simulink model "Gearbox_SLX"  (R2019b)
settings: Solver=VariableStepAuto  StartTime=0.0  StopTime=10.0  RelTol=1e-3
values from neighbouring files (symbols this model uses):
  b_mc = 1*(Nm/rad)    (= 1)    [Gearbox_SLX_m.m]
  J_mc = 1*kg*meters^2    (= 1)    [Gearbox_SLX_m.m]
  K_c = 10^7*(Newton/meters)    (= 10000000)    [Gearbox_SLX_m.m]
  P_2_0 = 0    [Gearbox_SLX_m.m]
  r_1 = 1*cm    (= 0.01)    [Gearbox_SLX_m.m]
  r_2 = 9.7*cm    (= 0.097)    [Gearbox_SLX_m.m]
  T_m_0 = 20*Nm    (= 20)    [Gearbox_SLX_m.m]
  Ts = Tfin/Nr_Ts_Points    (= 0.0025)    [Gearbox_SLX_m.m]
  W_w_0 = 0*Nm    (= 0)    [Gearbox_SLX_m.m]
  x_5_0 = 0    [Gearbox_SLX_m.m]
settings Model: Creator=Luca  LastModifiedBy=giaco
settings DataIOCC: ReturnWorkspaceOutputs=off
settings DebuggingCC: ArithmeticOperatorsInVariantConditions=warning
settings SFSimCC: SimUseLocalCustomCode=off  CustomCodeUndefinedFunction=UseInterfaceOnly
settings RTWCC: RTWUseLocalCustomCode=off

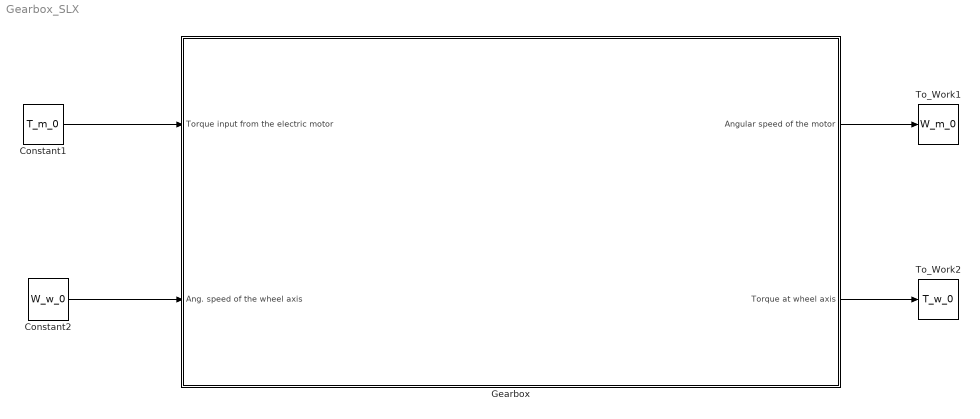
== system Gearbox_SLX ==
  Constant1 : Constant  Value=T_m_0
  Constant2 : Constant  Value=W_w_0
  Gearbox : Subsystem
  To_Work1 : ToWorkspace  VariableName=W_m_0  SampleTime=Ts
      settings: MaxDataPoints=10000
  To_Work2 : ToWorkspace  VariableName=T_w_0  SampleTime=Ts
      settings: MaxDataPoints=10000
  wires:
  Constant1/1 -> Gearbox/1(Torque input from the electric motor)
  Gearbox/1(Angular speed of the motor) -> To_Work1/1
  Gearbox/2(Torque at wheel axis) -> To_Work2/1
  Constant2/1 -> Gearbox/2(Ang. speed of the wheel axis)

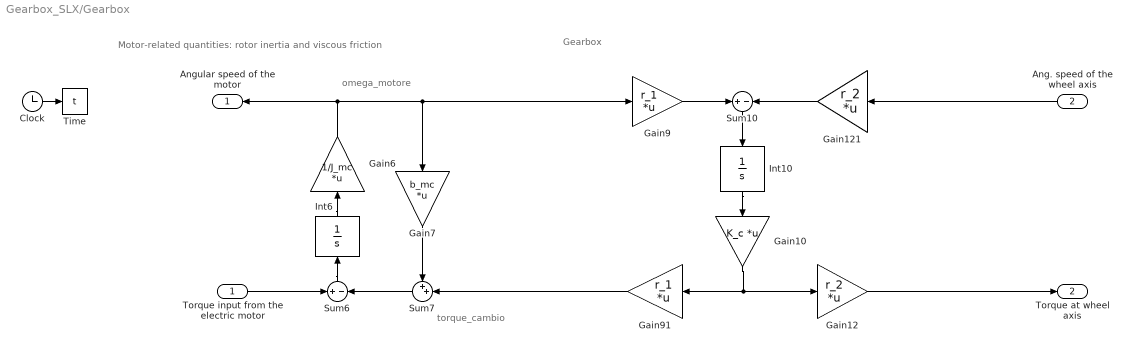
== system Gearbox_SLX/Gearbox ==
  note: omega_motore
  note: torque_cambio
  note: Motor-related quantities: rotor inertia and viscous friction
  note: Gearbox
  Torque input from the electric motor : Inport
  Ang. speed of the wheel axis : Inport  Port=2
  Clock : Clock
  Gain10 : Gain  Gain=K_c  Multiplication=Matrix(K*u)  SaturateOnIntegerOverflow=on  OutDataTypeStr=Inherit: Same as input  ParamDataTypeStr=Inherit: Same as input
  Gain12 : Gain  Gain=r_2  Multiplication=Matrix(K*u)  SaturateOnIntegerOverflow=on  OutDataTypeStr=Inherit: Same as input  ParamDataTypeStr=Inherit: Same as input
  Gain121 : Gain  Gain=r_2  Multiplication=Matrix(K*u)  SaturateOnIntegerOverflow=on  OutDataTypeStr=Inherit: Same as input  ParamDataTypeStr=Inherit: Same as input
  Gain6 : Gain  Gain=1/J_mc  Multiplication=Matrix(K*u)  SaturateOnIntegerOverflow=on  OutDataTypeStr=Inherit: Same as input  ParamDataTypeStr=Inherit: Same as input
  Gain7 : Gain  Gain=b_mc  Multiplication=Matrix(K*u)  SaturateOnIntegerOverflow=on  OutDataTypeStr=Inherit: Same as input  ParamDataTypeStr=Inherit: Same as input
  Gain9 : Gain  Gain=r_1  Multiplication=Matrix(K*u)  SaturateOnIntegerOverflow=on  OutDataTypeStr=Inherit: Same as input  ParamDataTypeStr=Inherit: Same as input
  Gain91 : Gain  Gain=r_1  Multiplication=Matrix(K*u)  SaturateOnIntegerOverflow=on  OutDataTypeStr=Inherit: Same as input  ParamDataTypeStr=Inherit: Same as input
  Int10 : Integrator  InitialCondition=x_5_0
  Int6 : Integrator  InitialCondition=P_2_0
  Sum10 : Sum  Inputs=+|-  SaturateOnIntegerOverflow=on  InputSameDT=on  OutDataTypeStr=Inherit: Same as first input
  Sum6 : Sum  Inputs=+|-  SaturateOnIntegerOverflow=on  InputSameDT=on  OutDataTypeStr=Inherit: Same as first input
  Sum7 : Sum  Inputs=++|  SaturateOnIntegerOverflow=on  InputSameDT=on  OutDataTypeStr=Inherit: Same as first input
  Time : ToWorkspace  VariableName=t  SampleTime=Ts
      settings: MaxDataPoints=10000
  Angular speed of the motor : Outport  VectorParamsAs1DForOutWhenUnconnected=off
  Torque at wheel axis : Outport  Port=2  VectorParamsAs1DForOutWhenUnconnected=off
  wires:
  Clock/1 -> Time/1
  Torque input from the electric motor/1 -> Sum6/1
  Sum7/1 -> Sum6/2
  Sum6/1 -> Int6/1
  Int6/1 -> Gain6/1
  Gain7/1 -> Sum7/1
  Gain91/1 -> Sum7/2
  Gain6/1 -> Angular speed of the motor/1, Gain7/1, Gain9/1
  Gain121/1 -> Sum10/2
  Gain9/1 -> Sum10/1
  Int10/1 -> Gain10/1
  Sum10/1 -> Int10/1
  Gain10/1 -> Gain12/1, Gain91/1
  Gain12/1 -> Torque at wheel axis/1
  Ang. speed of the wheel axis/1 -> Gain121/1
